simulink model "SPWM"  (R2021a)
settings: Solver=VariableStepAuto  StartTime=0.0  StopTime=1  RelTol=1e-3
undefined symbols (not defined in the file): Fm
libraries: spsSawtoothGeneratorLib x1
settings Model: Creator=SARTHAK  LastModifiedBy=smita
settings SolverCC: AlgebraicLoopSolver=TrustRegion
settings DebuggingCC: SFMachineParentedDataDiag=warning

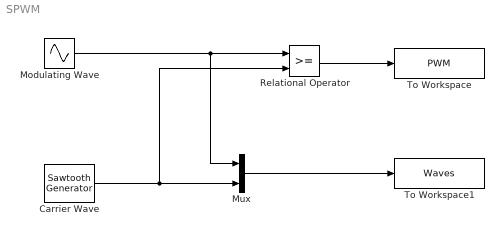
== system SPWM ==
  Carrier Wave : spsSawtoothGeneratorLib/Sawtooth Generator  Freq=Fc  Phase=180  Ts=0
  Modulating Wave : Sin  Frequency=2*pi*Fm  SampleTime=1/10000
  Mux : Mux  Inputs=2
  Relational Operator : RelationalOperator  OutDataTypeStr=boolean  RndMeth=Simplest
  To Workspace : ToWorkspace  VariableName=PWM  SaveFormat=Timeseries  SampleTime=-1
  To Workspace1 : ToWorkspace  VariableName=Waves  SaveFormat=Timeseries  SampleTime=-1
  wires:
  Relational Operator/1 -> To Workspace/1
  Mux/1 -> To Workspace1/1
  Modulating Wave/1 -> Mux/1, Relational Operator/1
  Carrier Wave/1 -> Relational Operator/2, Mux/2
